simulink model "blankpage"  (R2018a)
settings: Solver=ode4  StartTime=0.0  StopTime=endTime  FixedStep=timeStep  RelTol=1e-3
model workspace (MAT data in the model file):
  endTime = 12
  propulsion : struct (value not decoded)
  simInput : struct (value not decoded)
  timeProfile = [0 0.001 0.002 0.003 0.004 0.005 0.006 0.007 0.008 0.009 0.01 0.011 ... (12001 elements, 1x12001)]
  timeStep = 0.001
symbols that are objects in the model workspace (value not decoded): simInput
libraries: elementsLibrary x1
(part 2 of 2)

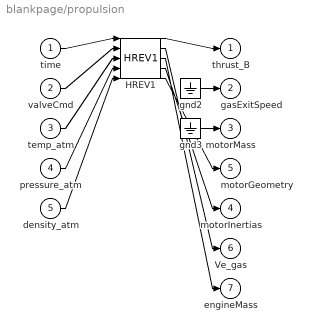
== system blankpage/propulsion ==
  time : Inport
  valveCmd : Inport  Port=2
  temp_atm : Inport  Port=3
  pressure_atm : Inport  Port=4
  "density_atm " : Inport  Port=5
  HREV1 : elementsLibrary/HREV1  propulsion=propulsion
  gnd2 : Ground
  gnd3 : Ground
  thrust_B : Outport
  gasExitSpeed : Outport  Port=2
  motorMass : Outport  Port=3
  motorInertias : Outport  Port=4
  motorGeometry : Outport  Port=5
  Ve_gas : Outport  Port=6
  engineMass : Outport  Port=7
  wires:
  time/1 -> HREV1/1
  valveCmd/1 -> HREV1/2
  temp_atm/1 -> HREV1/3
  pressure_atm/1 -> HREV1/4
  "density_atm "/1 -> HREV1/5
  HREV1/1 -> thrust_B/1
  HREV1/2 -> Ve_gas/1
  HREV1/3 -> engineMass/1
  HREV1/4 -> motorInertias/1
  HREV1/5 -> motorGeometry/1
  gnd2/1 -> gasExitSpeed/1
  gnd3/1 -> motorMass/1
